simulink model "A3_1_VorKin"  (R2023a)
settings: Solver=VariableStepAuto  StartTime=0.0  StopTime=10.0  RelTol=1e-3
values from neighbouring files (symbols this model uses):
  params = [l2 l3]    [A3_1_init_VorKin.m]    (also in A3_2_init_InvKin.m; init_InvKin.m)
settings Model: Creator=Flo  LastModifiedBy=Flo

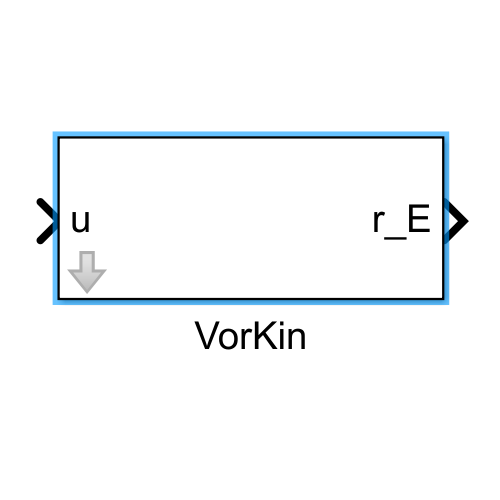
[thumbnail: Simulink's stored preview of the top-level diagram]
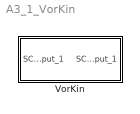
== system A3_1_VorKin ==
  VorKin : Subsystem  mask{SC_param_0=params}
      mask prompts: SC_param_0 "params"
      mask Display:
      | port_label('input', 1, 'u');
      | port_label('output', 1, 'r_E');

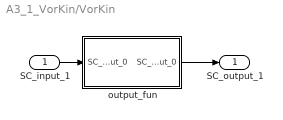
== system A3_1_VorKin/VorKin ==
  SC_input_1 : Inport
  output_fun : MATLAB Function  TreatAsAtomicUnit=on
  SC_output_1 : Outport
  wires:
  SC_input_1/1 -> output_fun/1(SC_input_0)
  output_fun/1(SC_output_0) -> SC_output_1/1

== matlab function A3_1_VorKin/VorKin/output_fun ==
  data: SC_input_0 input size=[3]; SC_output_0 output size=[3]; SC_param_0 parameter size=[2]
function SC_output_0  = y_fun(SC_input_0, SC_param_0)
    SC_output_0 = zeros(3,1);
    t1 = SC_input_0(1);
    t2 = cos(t1);
    t3 = SC_input_0(3);
    t4 = cos(t3);
    t5 = SC_param_0(2);
    t7 = SC_input_0(2);
    t8 = sin(t7);
    t9 = SC_param_0(1);
    t11 = t4 * t5 + t8 * t9;
    SC_output_0(1) = t11 * t2;
    t12 = sin(t3);
    t14 = cos(t7);
    SC_output_0(2) = t12 * t5 + t14 * t9;
    t16 = sin(t1);
    SC_output_0(3) = t16 * t11;
end
